simulink model "saturation_mdl"  (R2013b)
settings: Solver=ode45  StartTime=0.0  StopTime=10.0  RelTol=1e-3
libraries: cstblocks x4
settings Model: Creator=daniw  LastModifiedBy=daniw

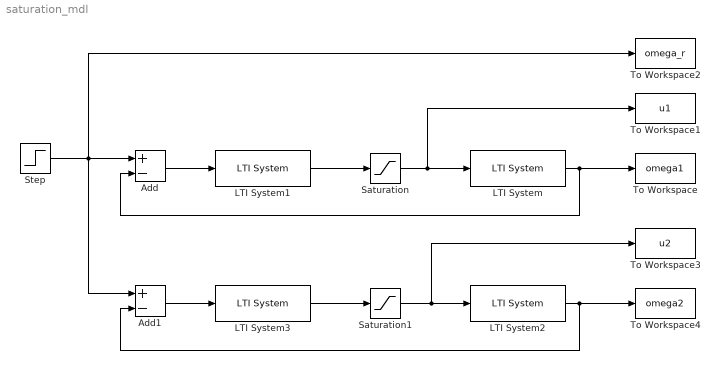
== system saturation_mdl ==
  Add : Sum  Inputs=+-
  Add1 : Sum  Inputs=+-
  LTI System : cstblocks/LTI System  sys=G11_man  IC=[]
  LTI System1 : cstblocks/LTI System  sys=C_PI  IC=[]
  LTI System2 : cstblocks/LTI System  sys=G12_man  IC=[]
  LTI System3 : cstblocks/LTI System  sys=C_PI  IC=[]
  Saturation : Saturate  UpperLimit=24  LowerLimit=-24
  Saturation1 : Saturate  UpperLimit=24  LowerLimit=-24
  Step : Step  After=2500  SampleTime=0
  To Workspace : ToWorkspace  VariableName=omega1  SampleTime=-1  SaveFormat=Structure With Time
  To Workspace1 : ToWorkspace  VariableName=u1  SampleTime=-1  SaveFormat=Structure With Time
  To Workspace2 : ToWorkspace  VariableName=omega_r  SampleTime=-1  SaveFormat=Structure With Time
  To Workspace3 : ToWorkspace  VariableName=u2  SampleTime=-1  SaveFormat=Structure With Time
  To Workspace4 : ToWorkspace  VariableName=omega2  SampleTime=-1  SaveFormat=Structure With Time
  wires:
  Step/1 -> Add1/1, To Workspace2/1, Add/1
  Add/1 -> LTI System1/1
  LTI System1/1 -> Saturation/1
  Saturation/1 -> To Workspace1/1, LTI System/1
  LTI System/1 -> To Workspace/1, Add/2
  Add1/1 -> LTI System3/1
  LTI System3/1 -> Saturation1/1
  Saturation1/1 -> To Workspace3/1, LTI System2/1
  LTI System2/1 -> To Workspace4/1, Add1/2
